simulink model "ThreeBitDigitalMultiplier"  (R2020b)
settings: Solver=VariableStepAuto  StartTime=0.0  StopTime=10.0  RelTol=1e-3
settings Model: Creator=mluser  LastModifiedBy=mluser

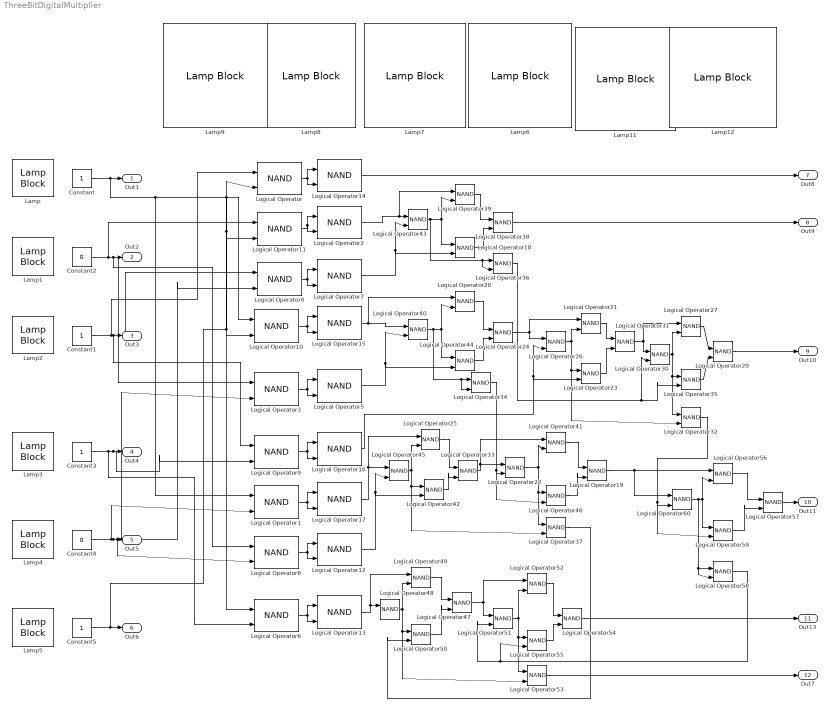
== system ThreeBitDigitalMultiplier ==
  Constant{,1,3,5} (4 alike) : Constant
  Constant2 : Constant  Value=0
  Constant4 : Constant  Value=0
  Lamp{,1..9,11..12} (12 alike) : LampBlock
  Logical Operator{,1..27,29..60} (60 alike) : Logic  Operator=NAND  IconShape=distinctive  AllPortsSameDT=off  OutDataTypeStr=boolean
  Out1 : Outport
  Out2 : Outport  Port=2
  Out3 : Outport  Port=3
  Out4 : Outport  Port=4
  Out5 : Outport  Port=5
  Out6 : Outport  Port=6
  Out8 : Outport  Port=7
  Out9 : Outport  Port=8
  Out10 : Outport  Port=9
  Out11 : Outport  Port=10
  Out13 : Outport  Port=11
  Out7 : Outport  Port=12
  wires:
  Constant4/1 -> Logical Operator1/2, Logical Operator3/2, Logical Operator4/2, Logical Operator8/2, Out5/1
  Constant/1 -> Logical Operator6/1, Logical Operator10/1, Logical Operator1/1, Out1/1
  Constant2/1 -> Logical Operator11/1, Logical Operator8/1, Out2/1, Logical Operator3/1
  Constant1/1 -> Logical Operator/1, Logical Operator4/1, Logical Operator9/1, Out3/1
  Constant3/1 -> Logical Operator9/2, Out4/1, Logical Operator6/2
  Constant5/1 -> Logical Operator10/2, Logical Operator11/2, Logical Operator/2, Out6/1
  Logical Operator/1 -> Logical Operator14/1, Logical Operator14/2
  Logical Operator11/1 -> Logical Operator2/1, Logical Operator2/2
  Logical Operator4/1 -> Logical Operator7/1, Logical Operator7/2
  Logical Operator10/1 -> Logical Operator15/1, Logical Operator15/2
  Logical Operator3/1 -> Logical Operator5/1, Logical Operator5/2
  Logical Operator9/1 -> Logical Operator16/1, Logical Operator16/2
  Logical Operator1/1 -> Logical Operator17/1, Logical Operator17/2
  Logical Operator8/1 -> Logical Operator12/1, Logical Operator12/2
  Logical Operator6/1 -> Logical Operator13/1, Logical Operator13/2
  Logical Operator2/1 -> Logical Operator39/1, Logical Operator43/1
  Logical Operator7/1 -> Logical Operator18/2, Logical Operator43/2
  Logical Operator43/1 -> Logical Operator36/2, Logical Operator36/1, Logical Operator39/2, Logical Operator18/1
  Logical Operator39/1 -> Logical Operator38/1
  Logical Operator18/1 -> Logical Operator38/2
  Logical Operator15/1 -> Logical Operator20/1, Logical Operator40/1
  Logical Operator5/1 -> Logical Operator44/2, Logical Operator40/2
  Logical Operator40/1 -> Logical Operator34/2, Logical Operator34/1, Logical Operator44/1, Logical Operator20/2
  Logical Operator20/1 -> Logical Operator24/1
  Logical Operator44/1 -> Logical Operator24/2
  Logical Operator42/1 -> Logical Operator33/2
  Logical Operator46/1 -> Logical Operator19/2
  Logical Operator12/1 -> Logical Operator42/2, Logical Operator45/2
  Logical Operator17/1 -> Logical Operator25/1, Logical Operator45/1
  Logical Operator45/1 -> Logical Operator37/2, Logical Operator42/1, Logical Operator25/2
  Logical Operator25/1 -> Logical Operator33/1
  Logical Operator33/1 -> Logical Operator22/1, Logical Operator41/1
  Logical Operator22/1 -> Logical Operator46/1, Logical Operator37/1, Logical Operator41/2
  Logical Operator41/1 -> Logical Operator19/1
  Logical Operator34/1 -> Logical Operator46/2, Logical Operator22/2
  Logical Operator24/1 -> Logical Operator21/1, Logical Operator26/1
  Logical Operator26/1 -> Logical Operator32/2, Logical Operator23/1, Logical Operator21/2
  Logical Operator16/1 -> Logical Operator26/2, Logical Operator23/2
  Logical Operator23/1 -> Logical Operator31/2
  Logical Operator21/1 -> Logical Operator31/1
  Logical Operator31/1 -> Logical Operator30/1, Logical Operator27/1
  Logical Operator30/1 -> Logical Operator32/1, Logical Operator35/1, Logical Operator27/2
  Logical Operator35/1 -> Logical Operator29/2
  Logical Operator27/1 -> Logical Operator29/1
  Logical Operator36/1 -> Logical Operator30/2, Logical Operator35/2
  Logical Operator47/1 -> Logical Operator52/1, Logical Operator51/1
  Logical Operator13/1 -> Logical Operator49/1, Logical Operator48/1
  Logical Operator48/1 -> Logical Operator49/2, Logical Operator53/2, Logical Operator50/1
  Logical Operator37/1 -> Logical Operator50/2
  Logical Operator52/1 -> Logical Operator54/1
  Logical Operator55/1 -> Logical Operator54/2
  Logical Operator51/1 -> Logical Operator52/2, Logical Operator53/1, Logical Operator55/1
  Logical Operator50/1 -> Logical Operator47/2
  Logical Operator49/1 -> Logical Operator47/1
  Logical Operator32/1 -> Logical Operator59/2, Logical Operator60/2
  Logical Operator60/1 -> Logical Operator58/2, Logical Operator58/1, Logical Operator56/2, Logical Operator59/1
  Logical Operator59/1 -> Logical Operator57/2
  Logical Operator56/1 -> Logical Operator57/1
  Logical Operator19/1 -> Logical Operator60/1, Logical Operator56/1
  Logical Operator14/1 -> Out8/1
  Logical Operator38/1 -> Out9/1
  Logical Operator29/1 -> Out10/1
  Logical Operator57/1 -> Out11/1
  Logical Operator53/1 -> Out7/1
  Logical Operator54/1 -> Out13/1
  Logical Operator58/1 -> Logical Operator55/2, Logical Operator51/2
